simulink model "pacing_and_sensing_unit"  (R2023b)
settings: Solver=FixedStepAuto  StartTime=0.0  StopTime=10.0  FixedStep=1e-3  RelTol=1e-3  EnableMultiTasking=on
undefined symbols (not defined in the file): D0, D1, D13, D3, D6, D8, PTA0, PTA1, PTC16, PTC17, PTC2, PTD1
libraries: frdmk64flib x6
settings Model: ExtModeTrigDuration=5  Creator=haley  LastModifiedBy=stivb
settings OptimizationCC: EnhancedBackFolding=on  PassReuseOutputArgsAs=Individual arguments  ZeroExternalMemoryAtStartup=off  ZeroInternalMemoryAtStartup=off  MaxStackSize=64  OptimizeBlockOrder=speed  DifferentSizesBufferReuse=on  OptimizationCustomize=off  EfficientTunableParamExpr=on
settings DebuggingCC: ParameterTunabilityLossMsg=error
settings HardwareCC: ProdBitPerPointer=32  ProdBitPerSizeT=32  ProdBitPerPtrDiffT=32  ProdLargestAtomicInteger=Long  ProdLargestAtomicFloat=Double  ProdWordSize=32  ProdHWDeviceType=ARM Compatible->ARM Cortex
settings SFSimCC: MATLABDynamicMemAlloc=off
settings RTWCC: Description=Embedded Coder  SystemTargetFile=ert.tlc  HardwareBoard=NXP FRDM-K64F  TLCOptions="-aInlineSetEventsForThisBaseRateFcn=TLC_FALSE -aSuppressMultiTaskScheduler=TLC_FALSE  -aRateBasedStepFcn=0"  TemplateMakefile=ert_default_tmf  Toolchain=GNU Tools for ARM Embedded Processors
settings CodeAppCC: ForceParamTrailComments=on  IgnoreCustomStorageClasses=off  OperatorAnnotations=on  SimulinkDataObjDesc=on  SFDataObjDesc=on  InsertBlockDesc=on
settings ERTTargetCC: ExtModeTransport=4  ExtModeMexFile=sendToCommService

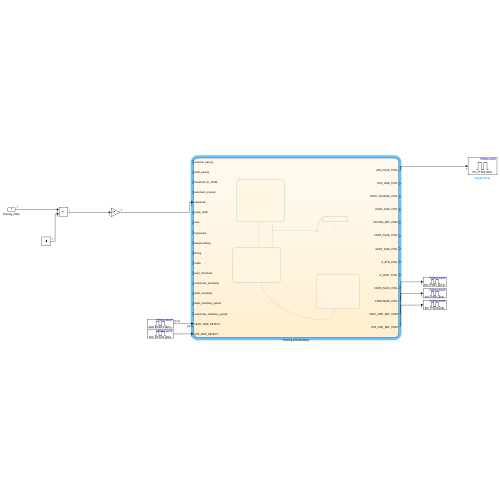
[thumbnail: Simulink's stored preview of the top-level diagram]
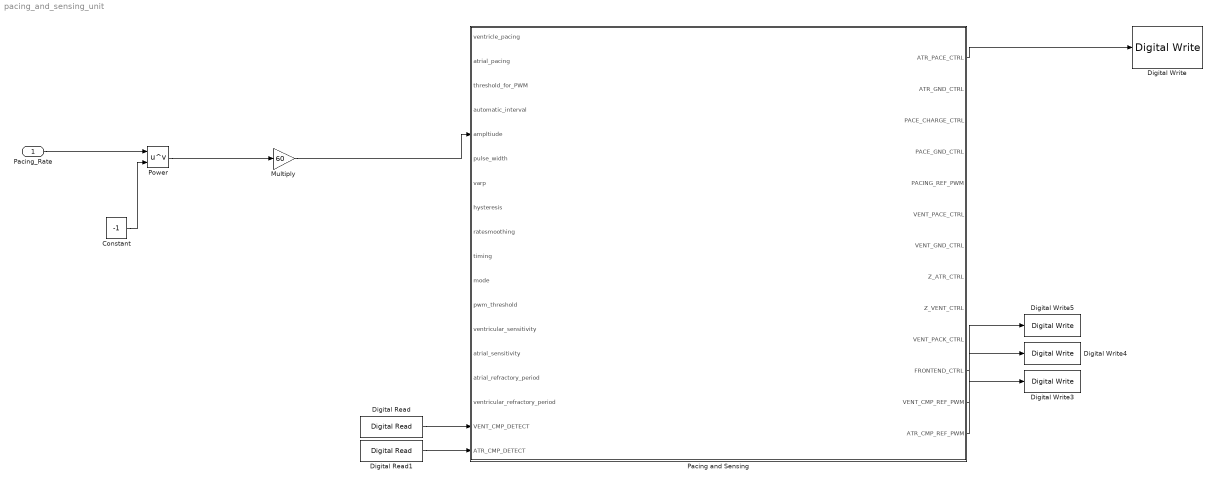
== system pacing_and_sensing_unit ==
  Pacing_Rate : Inport
  Constant : Constant  Value=-1
  Digital Read : frdmk64flib/Digital Read  Whichpin=PTC17 (D1)  SampleTime=-1
  Digital Read1 : frdmk64flib/Digital Read  Whichpin=PTC16 (D0)  SampleTime=-1
  Digital Write : frdmk64flib/Digital Write  Whichpin=PTA0 (D8)
  Digital Write3 : frdmk64flib/Digital Write  Whichpin=PTC2 (D6)
  Digital Write4 : frdmk64flib/Digital Write  Whichpin=PTA1 (D3)
  Digital Write5 : frdmk64flib/Digital Write  Whichpin=PTD1 (D13)
  Multiply : Gain  Gain=60
  Pacing and Sensing : Stateflow chart  TreatAsAtomicUnit=on
  Power : Math  Operator=pow
  wires:
  Pacing and Sensing/1(ATR_PACE_CTRL) -> Digital Write/1
  Power/1 -> Multiply/1
  Multiply/1 -> Pacing and Sensing/5(ampltiude)
  Constant/1 -> Power/2
  Pacing_Rate/1 -> Power/1
  Pacing and Sensing/11(FRONTEND_CTRL) -> Digital Write5/1
  Pacing and Sensing/12(VENT_CMP_REF_PWM) -> Digital Write4/1
  Pacing and Sensing/13(ATR_CMP_REF_PWM) -> Digital Write3/1
  Digital Read/1 -> Pacing and Sensing/17(VENT_CMP_DETECT)
  Digital Read1/1 -> Pacing and Sensing/18(ATR_CMP_DETECT)

== stateflow chart pacing_and_sensing_unit/Pacing and Sensing ==
  state Charge_Discharge_C22
    entry:
    %Charge
    ATR_PACE_CTRL = 0;
    VENT_PACE_CTRL = 0;
    PACE_CHARGE_CTRL = 1;
    PACING_REF_PWM = pwm_threshold; %percentage
    %Discharge
    PACE_GND_CTRL = 1;
    VENT_PACK_CTRL = 0;
    Z_ATR_CTRL = 0;
    Z_VENT_CTRL = 0;
    ATR_PACE_CTRL = 0;
    ATR_GND_CTRL = atrial_pacing;
    VENT_GND_CTRL= ventricle_pacing;
  state AtrialSensing
    detection = ATR_CMP_DETECT;
  note: Enter sensing state
  note: If not in sensing, continue pacing at automatic interval
  state ChargeC21
    %Creates the leading edge and sends pulse for X amount of time
    entry:
    PACE_CHARGE_CTRL = 0;
    PACE_GND_CTRL = 1;
    ATR_PACE_CTRL = atrial_pacing;
    ATR_GND_CTRL = 0;
    Z_ATR_CTRL = 0;
    Z_VENT_CTRL = 0;
    VENT_GND_CTRL = 0;
    VENT_PACE_CTRL = ventricle_pacing;
    %Recharge pulse is the current in the opposite direction due to C21
  state Sensing
    entry:
    % activate the sensing circuitry
    FRONTEND_CTRL = 1;
  (default) -> Charge_Discharge_C22
  (junction 103) -> AtrialSensing : [atrial_sensitivity ~= 0]
  ChargeC21 -> Charge_Discharge_C22 : after(pulse_width, sec)
  Charge_Discharge_C22 -> (junction 67)
  AtrialSensing -> ? : [detection == 1]
  (junction 67) -> (junction 103) [order 1] : [mode == 1]
  (junction 67) -> ChargeC21 [order 2] : [mode == 0 && after(automatic_interval, sec)]
  Sensing -> ChargeC21 : %statement where the timer has elasped
  data: ventricle_pacing input; atrial_pacing input; threshold_for_PWM input; ATR_PACE_CTRL output; ATR_GND_CTRL output; PACE_CHARGE_CTRL output; PACE_GND_CTRL output; PACING_REF_PWM output; VENT_PACE_CTRL output; VENT_GND_CTRL output; Z_ATR_CTRL output; Z_VENT_CTRL output; automatic_interval input; ampltiude input; pulse_width input; varp input; hysteresis input boolean; ratesmoothing input; timing input; mode input; pwm_threshold input; VENT_PACK_CTRL output; FRONTEND_CTRL output boolean; VENT_CMP_REF_PWM output boolean; ATR_CMP_REF_PWM output boolean; ventricular_sensitivity input double; atrial_sensitivity input double; atrial_refractory_period input uint32; ventricular_refractory_period input uint32; VENT_CMP_DETECT input boolean; ATR_CMP_DETECT input boolean
